simulink model "VSC_Simulink"  (R2019b)
settings: Solver=FixedStepDiscrete  StartTime=0.0  StopTime=Inf  FixedStep=T_pwm  MaxStep=1e-4  EnableMultiTasking=on
model workspace (MAT data in the model file):
  Control_P = 0
  Control_PI = 0
  I_integral = 0
  Id_pulse = 0
  Id_ref_const = 0
  Id_simulink = 0
  Id_sin = 0
  Iq_pulse = 0
  Iq_ref_const = 0
  Iq_simulink = 0
  Iq_sin = 0
  K_integral = 0
  K_proporcional = 0
  SELDACB = 0
  SELPWM4A = 0
  SELPWM4B = 0
  SELPWM5A = 0
  SELPWM5B = 0
  SELPWM6A = 0
  SELPWM6B = 0
  a_d = 0
  a_q = 0
  b_integral = 0
  b_proporcional = 0
  open = 0
  open_Id = 0
  open_Iq = 0
  open_control = 0
values from neighbouring files (symbols this model uses):
  Dec = 1    [Sotfware_Matlab.m]
  Frecuencia_Red = 50    [Sotfware_Matlab.m]
  Ib = 2.5    [Sotfware_Matlab.m]
  Ireg_PI = tan((90 + Fc_pi)*pi/180)/wo_pi    [Sotfware_Matlab.m]
  Kreg_P = 1/AP    [Sotfware_Matlab.m]
  Kreg_PI = Ac_pi*Ireg_PI*wo_pi / sqrt(1 + (Ireg_PI*wo_pi)^2)    [Sotfware_Matlab.m]
  Lpu = X_ind/ Lb    [Sotfware_Matlab.m]
  T_pwm = 1/Freq_Conmutacion    (= 0.0001)    [Sotfware_Matlab.m]
  TimerPeriod = Freq_Clock/(Freq_Conmutacion*4)    (= 5000)    [Sotfware_Matlab.m]
  Ub = 0.61*Vdc / sqrt(3)    [Sotfware_Matlab.m]
  w1pu = 1    [Sotfware_Matlab.m]
undefined symbols (not defined in the file or in its folder): Down, GPTRIP1SEL, GPTRIP2SEL, TZ1, TZ2, Up
libraries: c2802xlib x12, c2837xDlib x10, eeTransforms x2, simulink x2
(part 1 of 2)
settings Model: SimulationMode=external  ExtModeTrigDuration=8  TunableVars=SELPWM4A,SELPWM4B  TunableVarsStorageClass=Auto,Auto  TunableVarsTypeQualifier=const,const  ParameterArgumentNames=Control_P,Control_PI,I_integral,Id_pulse,Id_ref_const,Id_simulink,Id_sin,Iq_pulse,Iq_ref_const,Iq_simulink,Iq_sin,K_integral,K_proporcional,SELDACB,SELPWM4A,SELPWM4B,SELPWM5A,SELPWM5B,SELPWM6A,SELPWM6B,a_d,a_q,b_integral,b_proporcional,open,open_Id,open_Iq,open_control  OrderedModelArguments=off  Creator=jorge  LastModifiedBy=jorge
settings OptimizationCC: DefaultUnderspecifiedDataType=single  EnhancedBackFolding=on  PassReuseOutputArgsAs=Individual arguments  MaxStackSize=512  OptimizeBlockOrder=speed  DifferentSizesBufferReuse=on  OptimizationCustomize=off  EfficientTunableParamExpr=on
settings DebuggingCC: ParameterTunabilityLossMsg=error
settings HardwareCC: ProdBitPerChar=16  ProdBitPerInt=16  ProdBitPerPointer=32  ProdBitPerSizeT=32  ProdBitPerPtrDiffT=32  ProdLargestAtomicInteger=Integer  ProdLargestAtomicFloat=None  ProdWordSize=16  ProdLongLongMode=on  ProdHWDeviceType=Texas Instruments->C2000
settings SFSimCC: MATLABDynamicMemAlloc=off  CustomCodeUndefinedFunction=UseInterfaceOnly
settings RTWCC: SystemTargetFile=ert.tlc  HardwareBoard=TI Delfino F28379D LaunchPad  TLCOptions=-aInlineSetEventsForThisBaseRateFcn=TLC_FALSE -aSuppressMultiTaskScheduler=TLC_FALSE -aRateBasedStepFcn=1  TemplateMakefile=ert_default_tmf  GenerateReport=on  Toolchain=Texas Instruments Code Composer Studio (C2000)  IncludeHyperlinkInReport=on  LaunchReport=on  GenerateTraceInfo=on  GenerateTraceReport=on  GenerateTraceReportSl=on  GenerateTraceReportSf=on  GenerateTraceReportEml=on
settings CodeAppCC: ForceParamTrailComments=on  IgnoreCustomStorageClasses=off  OperatorAnnotations=on  SimulinkDataObjDesc=on  SFDataObjDesc=on  InsertBlockDesc=on
settings ERTTargetCC: CodeReplacementLibrary=TI C28x  SupportContinuousTime=on

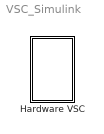
== system VSC_Simulink ==
  Hardware VSC : Subsystem  mask{Parameter1A=Id, Parameter1B=Id Referencia, Parameter2A=Iq, Parameter2B=Iq Referencia, ParameterDAC=Ángulo transformada de Park, Parameter3A=Va, Parameter3B=Ia, Id_simulink=1, Iq_simulink=1, refd=Pulsos, refq=Pulsos, control=Control PI, K_proporcional=Kreg_P, b_proporcional=1, K_integral=Kreg_PI*0.1, I_integral=Ireg_PI, b_integral=1, tipolazo=Lazo Cerrado, mandod=0, mandoq=0, acoplamiento=on}
      mask prompts: Parameter1A "PWM1A"; Parameter1B "PWM1B"; Parameter2A "PWM2A"; Parameter2B "PWM2B"; ParameterDAC "DAC - A"; Parameter3A "PWM3A"; Parameter3B "PWM3B"; Id_simulink "Id Referencia"; Iq_simulink "Iq Referencia"; refd "Forma de onda de referencia Id"; refq "Forma de onda de referencia Iq"; control "Selecciona el Control"; K_proporcional "K:"; b_proporcional "b:"; K_integral "K:"; I_integral "I:"; b_integral "b:"; tipolazo "Tipo de lazo"; mandod "Tensión de mando eje d  (md)"; mandoq "Tensión de mando eje q (mq)"
      mask init:
      | switch Parameter1A
      |     case 1
      |         SELPWM1A = 1;
      |     case 2
      |         SELPWM1A = 2;
      |     case 3
      |         SELPWM1A = 3;
      |     case 4
      |         SELPWM1A = 4;
      |     case 5
      |         SELPWM1A = 5;
      |     case 6
      |         SELPWM1A = 6;
      |     case 7
      |         SELPWM1A = 7;
      |     otherwise
      |         SELPWM1A = -1;
      | end
      | 
      | switch Parameter1B
      |     case 1
      |         SELPWM1B = 1;
      |     case 2
      |         SELPWM1B = 2;
      |     case 3
      |         SELPWM1B = 3;
      |     case 4
      |         SELPWM1B = 4;
      |     case 5
      |         SELPWM1B = 5;
      |     case 6
      |         SELPWM1B = 6;
      |     case 7
      |         SELPWM1B = 7;
      |     otherwise
      |         SELPWM1B = -1;
      | end
      | switch Parameter2A
      |     case 1
      |         SELPWM2A = 1;
      |     case 2
      |         SELPWM2A = 2;
      |     case 3
      |         SELPWM2A = 3;
      |     case 4
      |         SELPWM2A = 4;
      |     case 5
      |         SELPWM2A = 5;
      |     case 6
      |         SELPWM2A = 6;
      |     case 7
      |         SELPWM2A = 7;
      |     otherwise
      |         SELPWM2A = -1;
      | end
      | 
      | switch Parameter2B
      |     case 1
      |         SELPWM2B = 1;
      |     case 2
      |         SELPWM2B = 2;
      |     case 3
      |         SELPWM2B = 3;
      |     case 4
      |         SELPWM2B = 4;
      |     case 5
      |         SELPWM2B = 5;
      |     case 6
      |         SELPWM2B = 6;
      |     case 7
      |         SELPWM2B = 7;
      |     otherwise
      |         SELPWM2B = -1;
      | end
      | 
      | switch ParameterDAC
      |     case 1
      |         SELDACA = 1;
      |     case 2
      |         SELDACA = 2;
      |     case 3
      |         SELDACA = 3;
      |     case 4
      |         SELDACA = 4;
      |     case 5
      |         SELDACA = 5;
      |     case 6
      |         SELDACA = 6;
      |     case 7
      |         SELDACA = 7;
      |     otherwise
      |         SELDACA = -1;
      | end
      | switch Parameter3A
      |     case 1
      |         SELPWM3A = 8;
      |     case 2
      |         SELPWM3A = 9;
      |     case 3
      |         SELPWM3A = 10;
      |     case 4
      |         SELPWM3A = 11;
      |     case 5
      |         SELPWM3A = 12;
      |     case 6
      |         SELPWM3A = 13;
      |     otherwise
      |         SELPWM3A = -1;
      | end
      | switch Parameter3B
      |     case 1
      |         SELPWM3B = 8;
      |     case 2
      |         SELPWM3B = 9;
      |     case 3
      |         SELPWM3B = 10;
      |     case 4
      |         SELPWM3B = 11;
      |     case 5
      |         SELPWM3B = 12;
      |     case 6
      |         SELPWM3B = 13;
      |     otherwise
      |         SELPWM3B = -1;
      | end
      |        
      | switch refd
      |     case 1
      |         Id_ref_const = 1;
      |         Id_pulse = 0;
      |         Id_sin = 0;
      |     case 2
      |         Id_ref_const = 0;
      |         Id_pulse = 1;
      |         Id_sin = 0;        
      |     case 3
      |         Id_ref_const = 0;
      |         Id_pulse = 0;
      |         Id_sin = 1;
      | end
      | 
      | switch refq
      |     case 1
      |         Iq_ref_const = 1;
      |         Iq_pulse = 0;
      |         Iq_sin = 0;
      |     case 2
      |         Iq_ref_const = 0;
      |         Iq_pulse = 1;
      |         Iq_sin = 0;        
      |     case 3
      |         Iq_ref_const = 0;
      |         Iq_pulse = 0;
      |         Iq_sin = 1;
      | end
      | 
      | switch control
      |     case 1
      |         Control_P = 1;
      |         Control_PI = 0;
      |         I_integral = 1;
      |     case 2
      |         Control_P = 0;
      |         Control_PI = 1;
      | end
      | 
      | switch tipolazo
      |     case 1
      |         open = 0;
      |         a_d = mandod;
      |         a_q = mandoq;
      |     case 2
      |         open = 1;
      |         a_d = 0;
      |         a_q = 0;
      | end
      | 
      | if acoplamiento == 1
      |         open_Id = 1;
      |         open_Iq = 1;
      | else 
      |     open_Id = 0;
      |     open_Iq = 0;
      | end
      mask TypeOptions Parameter1A: Id | Iq | Id Referencia | Iq Referencia | md | mq | Ángulo transformada de Park
      mask TypeOptions Parameter1B: Id | Iq | Id Referencia | Iq Referencia | md | mq | Ángulo transformada de Park
      mask TypeOptions Parameter2A: Id | Iq | Id Referencia | Iq Referencia | md | mq | Ángulo transformada de Park
      mask TypeOptions Parameter2B: Id | Iq | Id Referencia | Iq Referencia | md | mq | Ángulo transformada de Park
      mask TypeOptions ParameterDAC: Id | Iq | Id Referencia | Iq Referencia | md | mq | Ángulo transformada de Park
      mask TypeOptions Parameter3A: Va | Vb | Vc | Ia | Ib | Ic
      mask TypeOptions Parameter3B: Va | Vb | Vc | Ia | Ib | Ic
      mask TypeOptions refd: Constante | Pulsos | Senoidal
      mask TypeOptions refq: Constante | Pulsos | Senoidal
      mask TypeOptions control: Control P | Control PI
      mask TypeOptions tipolazo: Lazo Abierto | Lazo Cerrado
      mask DialogControl Container7 Prompt: Salidas
      mask DialogControl Container9 Prompt: Referencias
      mask DialogControl Container12 Prompt: Controles
      mask DialogControl Container22 Prompt: Control Proporcional
      mask DialogControl Container24 Prompt: Control Proporcional - Integral
      mask DialogControl Container19 Prompt: Lazo
      mask DialogControl Container17 Prompt: Lazo Abierto
      mask DialogControl Container18 Prompt: Acoplamiento / Desacoplamiento
      mask Display: image('click.png'); % Use "Edit Image" on toolstrip to change.

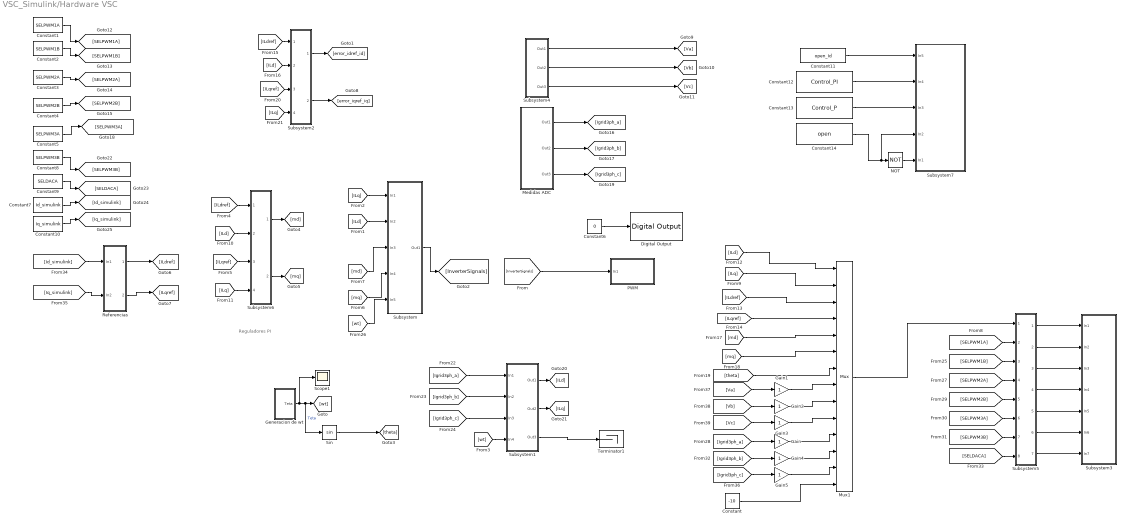
== system VSC_Simulink/Hardware VSC ==
  note: Reguladores PI
  Constant : Constant  Value=-10
  Constant1 : Constant  Value=SELPWM1A  SampleTime=-1
  Constant10 : Constant  Value=Iq_simulink  SampleTime=-1
  Constant11 : Constant  Value=open_Id  OutDataTypeStr=uint16  SampleTime=-1
  Constant12 : Constant  Value=Control_PI  SampleTime=-1
  Constant13 : Constant  Value=Control_P  SampleTime=-1
  Constant14 : Constant  Value=open  SampleTime=-1
  Constant2 : Constant  Value=SELPWM1B  SampleTime=-1
  Constant3 : Constant  Value=SELPWM2A  SampleTime=-1
  Constant4 : Constant  Value=SELPWM2B  SampleTime=-1
  Constant5 : Constant  Value=SELPWM3A
  Constant6 : Constant  Value=0  OutDataTypeStr=uint16  SampleTime=-1
  Constant7 : Constant  Value=Id_simulink  SampleTime=-1
  Constant8 : Constant  Value=SELPWM3B  SampleTime=-1
  Constant9 : Constant  Value=SELDACA  SampleTime=-1
  Digital Output : c2837xDlib/Digital Output  GPIO_Number=GPIO24~GPIO31  GPIO_Bit0=off  GPIO_BIT0_Toggle=off  GPIO_Bit1=off  GPIO_BIT1_Toggle=off  GPIO_Bit2=on  GPIO_BIT2_Toggle=on  GPIO_Bit3=off  GPIO_BIT3_Toggle=off  GPIO_Bit4=off  GPIO_BIT4_Toggle=off  GPIO_Bit5=off  GPIO_BIT5_Toggle=off  GPIO_Bit6=off  GPIO_BIT6_Toggle=off  GPIO_Bit7=off  GPIO_BIT7_Toggle=off
      settings: SourceProductName=Embedded Coder Support Package for Texas Instruments C2000 Processors  SourceProductBaseCode=TIC2000
  Gain{,1..5} (6 alike) : Gain  OutDataTypeStr=double
  Generacion de wt : Subsystem
  Medidas ADC : Subsystem
  Mux1 : Mux  Inputs=14
  NOT : Logic  Operator=NOT  IconShape=distinctive  AllPortsSameDT=off  OutDataTypeStr=boolean
  PWM : Subsystem
  Referencias : Subsystem
  Scope1 : Scope
  Sin : Trigonometry
  Subsystem : Subsystem
  Subsystem1 : Subsystem
  Subsystem2 : Subsystem
  Subsystem3 : Subsystem
  Subsystem4 : Subsystem
  Subsystem5 : Subsystem
  Subsystem6 : Subsystem
  Subsystem7 : Subsystem
  Terminator1 : Terminator
  wires:
  [Iq_simulink] -> Referencias/2(In2)
  [Id_simulink] -> Referencias/1(In1)
  Constant10/1 -> [Iq_simulink]
  Constant7/1 -> [Id_simulink]
  Constant9/1 -> [SELDACA]
  Constant4/1 -> [SELPWM2B]
  Constant5/1 -> [SELPWM3A]
  Constant3/1 -> [SELPWM2A]
  Constant2/1 -> [SELPWM1B]
  Constant1/1 -> [SELPWM1A]
  [SELDACA] -> Subsystem5/8(In8)
  [SELPWM3A] -> Subsystem5/6(In6)
  [SELPWM2B] -> Subsystem5/5(In5)
  [SELPWM2A] -> Subsystem5/4(In4)
  [SELPWM1B] -> Subsystem5/3(In3)
  [SELPWM1A] -> Subsystem5/2(In2)
  Mux1/1 -> Subsystem5/1(In1)
  Subsystem5/7(Out6) -> Subsystem3/7(In7)
  Subsystem5/6(Out5) -> Subsystem3/6(In6)
  Subsystem5/5(Out4) -> Subsystem3/5(In5)
  Subsystem5/4(Out3) -> Subsystem3/4(In4)
  Subsystem5/3(Out2) -> Subsystem3/3(In3)
  Subsystem5/2(Out1) -> Subsystem3/2(In2)
  Subsystem5/1(Out7) -> Subsystem3/1(In1)
  [md] -> Mux1/5
  [ILq] -> Mux1/2
  [ILd] -> Mux1/1
  [ILqref] -> Mux1/4
  [ILdref] -> Mux1/3
  Subsystem4/3(Out3) -> [Vc]
  Subsystem4/2(Out2) -> [Vb]
  Subsystem4/1(Out1) -> [Va]
  Constant6/1 -> Digital Output/1
  Subsystem2/2(Out2) -> [error_iqref_iq]
  Subsystem2/1(Out1) -> [error_idref_id]
  [ILq] -> Subsystem2/4(In4)
  [ILqref] -> Subsystem2/3(In3)
  [ILd] -> Subsystem2/2(In2)
  [ILdref] -> Subsystem2/1(In1)
  Sin/1 -> [theta]
  [md] -> Subsystem/3(In3)
  [mq] -> Subsystem/4(In4)
  Subsystem1/3(Out3) -> Terminator1/1
  Subsystem1/2(Out2) -> [ILq]
  [wt] -> Subsystem1/4(In4)
  [Igrid3ph_c] -> Subsystem1/3(In3)
  [Igrid3ph_b] -> Subsystem1/2(In2)
  [Igrid3ph_a] -> Subsystem1/1(In1)
  Subsystem1/1(Out1) -> [ILd]
  Referencias/2(Out2) -> [ILqref]
  Referencias/1(Out1) -> [ILdref]
  Subsystem/1(Out1) -> [InverterSignals]
  [wt] -> Subsystem/5(In5)
  [ILd] -> Subsystem/2(In2)
  [ILq] -> Subsystem/1(In1)
  Medidas ADC/3(Out3) -> [Igrid3ph_c]
  Medidas ADC/2(Out2) -> [Igrid3ph_b]
  Medidas ADC/1(Out1) -> [Igrid3ph_a]
  [InverterSignals] -> PWM/1(In1)
  Generacion de wt/1(Teta) -> Scope1/1, [wt], Sin/1  "Teta"
  Constant8/1 -> [SELPWM3B]
  [mq] -> Mux1/6
  [theta] -> Mux1/7
  [Igrid3ph_a] -> Gain/1
  Gain/1 -> Mux1/11
  Gain4/1 -> Mux1/12
  [Igrid3ph_b] -> Gain4/1
  [Igrid3ph_c] -> Gain5/1
  Gain5/1 -> Mux1/13
  [Vc] -> Gain3/1
  [Vb] -> Gain2/1
  [Va] -> Gain1/1
  Gain1/1 -> Mux1/8
  Gain2/1 -> Mux1/9
  Gain3/1 -> Mux1/10
  Constant/1 -> Mux1/14
  [SELPWM3B] -> Subsystem5/7(In7)
  Constant14/1 -> Subsystem7/4(In2), NOT/1
  Subsystem6/2(Out2) -> [mq]
  [ILdref] -> Subsystem6/1(In1)
  [ILqref] -> Subsystem6/3(In3)
  [ILq] -> Subsystem6/4(In4)
  [ILd] -> Subsystem6/2(In2)
  Subsystem6/1(Out1) -> [md]
  Constant13/1 -> Subsystem7/3(In3)
  Constant12/1 -> Subsystem7/2(In4)
  Constant11/1 -> Subsystem7/1(In5)
  NOT/1 -> Subsystem7/5(In1)

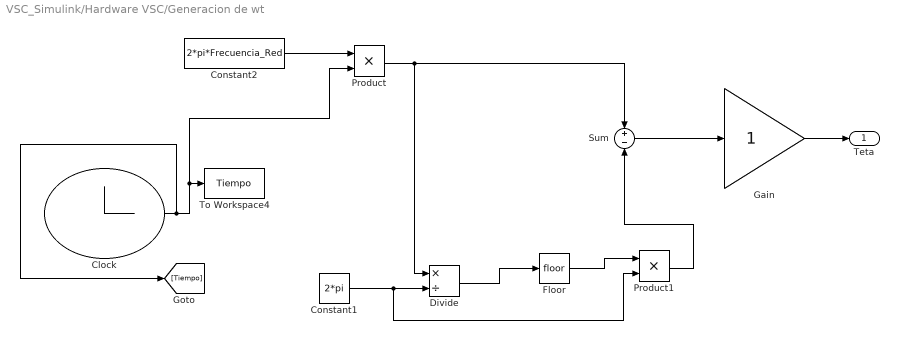
== system VSC_Simulink/Hardware VSC/Generacion de wt ==
  Clock : Clock
      settings: Decimation=100
  Constant1 : Constant  Value=2*pi  SampleTime=-1
  Constant2 : Constant  Value=2*pi*Frecuencia_Red  SampleTime=-1
  Divide : Product  Inputs=*/
  Floor : Rounding
  Gain : Gain
  Product : Product
  Product1 : Product
  Sum : Sum  Inputs=+-
  To Workspace4 : ToWorkspace  VariableName=Tiempo
  Teta : Outport  VectorParamsAs1DForOutWhenUnconnected=off
  wires:
  Product/1 -> Sum/1, Divide/1
  Constant1/1 -> Divide/2, Product1/2
  Product1/1 -> Sum/2
  Sum/1 -> Gain/1
  Divide/1 -> Floor/1
  Floor/1 -> Product1/1
  Constant2/1 -> Product/1
  Clock/1 -> To Workspace4/1, Product/2, [Tiempo]
  Gain/1 -> Teta/1

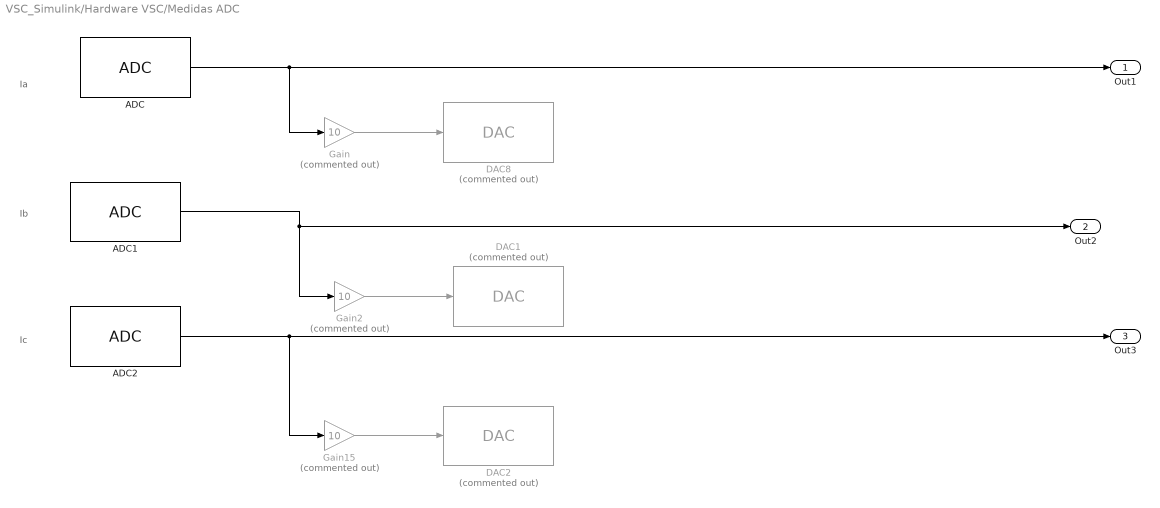
== system VSC_Simulink/Hardware VSC/Medidas ADC ==
  note: Ic
  note: Ia
  note: Ib
  ADC : c2802xlib/ADC  blkParamProc=C2000_Type4  ADCModule=C  samplingMode=Single sample mode  ADCResolution=12-bit (Single-ended input)  useSOC1=SOC8  useSOC2=SOC0_SOC1  SOCAcquisitionWindow=15  SOCTriggerSource=ePWM4_ADCSOCA  SOCInterruptTrigger=No ADCINT  Ts=-1  dType=uint16  postInterrupt=on  interruptSel=ADCINT1  ADCINTContinuous=on  endma=off  chdma=1  conv1=ADCINA0  conv2=ADCINA0 and ADCINB0  conv1_Type4=ADCIN4  conv2_Type4=ADCIN0 and ADCIN1
      settings: SourceProductName=Embedded Coder Support Package for Texas Instruments C2000 Processors
  ADC1 : c2802xlib/ADC  blkParamProc=C2000_Type4  ADCModule=B  samplingMode=Single sample mode  ADCResolution=12-bit (Single-ended input)  useSOC1=SOC9  useSOC2=SOC0_SOC1  SOCAcquisitionWindow=15  SOCTriggerSource=ePWM5_ADCSOCA  SOCInterruptTrigger=No ADCINT  Ts=-1  dType=uint16  postInterrupt=on  interruptSel=ADCINT1  ADCINTContinuous=on  endma=off  chdma=1  conv1=ADCINA0  conv2=ADCINA0 and ADCINB0  conv1_Type4=ADCIN4  conv2_Type4=ADCIN0 and ADCIN1
      settings: SourceProductName=Embedded Coder Support Package for Texas Instruments C2000 Processors
  ADC2 : c2802xlib/ADC  blkParamProc=C2000_Type4  ADCModule=A  samplingMode=Single sample mode  ADCResolution=12-bit (Single-ended input)  useSOC1=SOC10  useSOC2=SOC0_SOC1  SOCAcquisitionWindow=15  SOCTriggerSource=ePWM6_ADCSOCA  SOCInterruptTrigger=No ADCINT  Ts=-1  dType=uint16  postInterrupt=on  interruptSel=ADCINT1  ADCINTContinuous=on  endma=off  chdma=1  conv1=ADCINA0  conv2=ADCINA0 and ADCINB0  conv1_Type4=ADCIN4  conv2_Type4=ADCIN0 and ADCIN1
      settings: SourceProductName=Embedded Coder Support Package for Texas Instruments C2000 Processors
  DAC1 : c2837xDlib/DAC  Commented=on  channel=B  saturate=off
      settings: SourceProductName=Embedded Coder Support Package for Texas Instruments C2000 Processors  SourceProductBaseCode=TIC2000
  DAC2 : c2837xDlib/DAC  Commented=on  channel=B  saturate=off
      settings: SourceProductName=Embedded Coder Support Package for Texas Instruments C2000 Processors  SourceProductBaseCode=TIC2000
  DAC8 : c2837xDlib/DAC  Commented=on  channel=B  saturate=off
      settings: SourceProductName=Embedded Coder Support Package for Texas Instruments C2000 Processors  SourceProductBaseCode=TIC2000
  Gain : Gain  Commented=on  Gain=10
  Gain15 : Gain  Commented=on  Gain=10
  Gain2 : Gain  Commented=on  Gain=10
  Out1 : Outport  VectorParamsAs1DForOutWhenUnconnected=off
  Out2 : Outport  Port=2  VectorParamsAs1DForOutWhenUnconnected=off
  Out3 : Outport  Port=3  VectorParamsAs1DForOutWhenUnconnected=off
  wires:
  Gain/1 -> DAC8/1
  ADC2/1 -> Gain15/1, Out3/1
  ADC1/1 -> Gain2/1, Out2/1
  Gain2/1 -> DAC1/1
  Gain15/1 -> DAC2/1
  ADC/1 -> Gain/1, Out1/1

== system VSC_Simulink/Hardware VSC/PWM ==
  In1 : Inport
  Demux2 : Demux  Outputs=3
  ePWM1 : c2802xlib/ePWM  useModule=ePWM5  ePWMxLINKTBPRD=Not Linked  periodUnits=Clock cycles  timerSource=Specify via dialog  timerPeriod_clk=TimerPeriod  timerPeriod_sec=0.0001  tbshadow=Counter equals to zero  countingMode=Up-Down  phaseActiveEnable=Disable  phaseDirection=Count down after sync  phaseActive=0  synchronizationEnable=off  dcaevt1Sync=off  dcbevt1Sync=off  synchronizationOption=Disable  clockPrescale=1  HSclockPrescale=1  enswap=off  ePWMxAStatus=on  ePWMxAactionLogic1=Set  ePWMxAactionLogic2=Clear  ePWMxAactionLogic3=Clear  ePWMxAactionLogic4=Set  ePWMxAactionLogic5=Do nothing  ePWMxAactionLogic6=Do nothing  ePWMxALoadMode=Load on counter equals to zero (CTR=Zero)  ePWMxACSFenable=off  ePWMxACSFvalue=Forcing disable  ePWMxASFreload=Zero  ePWMxBStatus=off  ePWMxBactionLogic1=Set  ePWMxBactionLogic2=Clear  ePWMxBactionLogic3=Do nothing  ePWMxBactionLogic4=Do nothing  ePWMxBactionLogic5=Clear  ePWMxBactionLogic6=Set  ePWMxBLoadMode=Load on counter equals to zero (CTR=Zero)  ePWMxBCSFenable=off  ePWMxBCSFvalue=Forcing disable  ePWMxBSFreload=Zero  ePWNxBOutWay=off  ePWMxLINKCMPA=Not Linked  CMPAUnits=Clock cycles  CMPASource=Input port  CMPAValue_per=50  CMPAValue_clk=0  enCMPAshadow=Counter equals to zero  ePWMxLINKCMPB=Not Linked  CMPBUnits=Clock cycles  CMPBSource=Specify via dialog  CMPBValue_per=50  CMPBValue_clk=0  enCMPBshadow=Counter equals to zero  ePWMxLINKCMPC=Not Linked  CMPCUnits=Clock cycles  CMPCSource=Specify via dialog  CMPCValue_per=50  CMPCValue_clk=0  enCMPCshadow=Counter equals to zero  ePWMxLINKCMPD=Not Linked  CMPDUnits=Clock cycles  CMPDSource=Specify via dialog  CMPDValue_per=50  CMPDValue_clk=0  enCMPDshadow=Counter equals to zero  enableDBePWMxA=off  enableDBePWMxB=on  enhalfcycle=off  DBpolarity=Active high (AH)  DBedgeDelay=Negative  DBSource_ePWMxA=ePWMxA  DBSource_ePWMxB=ePWMxA  DBperiodSource=Specify via dialog  REDperiod=0  FEDperiod=0  adcstartModuleA=on  adcrequestEventA=Third event  adcstartEventA=Digital Compare Module A Event 1 start of conversion (DCAEVT1.soc)  adcstartEventA_type2=Counter equals to period (CTR=PRD)  adcstartModuleB=on  adcrequestEventB=Third event  adcstartEventB=Counter equals to zero (CTR=Zero)  adcstartEventB_type2=Counter equals to period (CTR=PRD)  intEn=off  intPrd=First event  intSel=Counter equals to zero (CTR=Zero)  intSel_type2=Counter equals to zero (CTR=Zero)  hrpe=off  enHRPWM=off  HRPWM_LoadMode=Counter equals to period (CTR=PRD)  HRPWM_CTLMode=Duty or Period control mode  HRPWM_EDGMode=Both edge  hrpeb=off  enHRPWMB=off  HRPWM_LoadModeB=Counter equals to zero (CTR=ZERO)  HRPWM_CTLModeB=Duty or Period control mode  HRPWM_EDGModeB=Both edge  enSFO=on  enautoconv=on  chopperEnable=off  chopperFrequency=1  chopperFirstwidth=1  chopperDuty=12.5%  tripZonesource=Specify via dialog  tzselOSHT1=off  tzselOSHT2=off  tzselOSHT3=off  tzselOSHDCAEV1=off  tzselOSHDCBEV1=off  tzselCBC1=off  tzselCBC2=off  tzselCBC3=off  tzselCBCDCAEV2=off  tzselCBCDCBEV2=off  tzselOSHT4=off  tzselOSHT5=off  tzselOSHT6=off  tzselCBC4=off  tzselCBC5=off  tzselCBC6=off  enTzOstIntr=off  enTzCbcIntr=off  enTzDCAEVT1Intr=off  enTzDCAEVT2Intr=off  enTzDCBEVT1Intr=off  enTzDCBEVT2Intr=off  ePWMxAforced=No action  ePWMxBforced=No action  DCAEVT1forced=No action  DCBEVT1forced=No action  DCAEVT2forced=No action  DCBEVT2forced=No action  dcah=Trip Zone 1 input (TZ1)  dcal=Trip Zone 2 input (TZ2)  dcbh=Trip Zone 1 input (TZ1)  dcbl=Trip Zone 2 input (TZ2)  dcah_type2=GPTRIP1SEL/(TZ1)  dcal_type2=GPTRIP2SEL/(TZ2)  dcbh_type2=GPTRIP1SEL/(TZ1)  dcbl_type2=GPTRIP2SEL/(TZ2)  gendcaevt1=Event disabled  gendcaevt2=Event disabled  gendcbevt1=Event disabled  gendcbevt2=Event disabled  dcaevt1src=DCAEVT1 with sync  dcaevt2src=DCAEVT2 with sync  dcbevt1src=DCBEVT1 with sync  dcbevt2src=DCBEVT2 with sync  pulsesel=Counter equals to zero (CTR=Zero)  blankinv=off  blankoffset=0  blankwidth=0  evsrcsel=Filtered version of DCAEVT1 (DCAEVT1FILT)  encape=off  PwmType=C2000_Type4
      settings: SourceProductName=Embedded Coder Support Package for Texas Instruments C2000 Processors
  ePWM2 : c2802xlib/ePWM  useModule=ePWM6  ePWMxLINKTBPRD=Not Linked  periodUnits=Clock cycles  timerSource=Specify via dialog  timerPeriod_clk=TimerPeriod  timerPeriod_sec=0.0001  tbshadow=Counter equals to zero  countingMode=Up-Down  phaseActiveEnable=Disable  phaseDirection=Count down after sync  phaseActive=0  synchronizationEnable=off  dcaevt1Sync=off  dcbevt1Sync=off  synchronizationOption=Disable  clockPrescale=1  HSclockPrescale=1  enswap=off  ePWMxAStatus=on  ePWMxAactionLogic1=Set  ePWMxAactionLogic2=Clear  ePWMxAactionLogic3=Clear  ePWMxAactionLogic4=Set  ePWMxAactionLogic5=Do nothing  ePWMxAactionLogic6=Do nothing  ePWMxALoadMode=Load on counter equals to zero (CTR=Zero)  ePWMxACSFenable=off  ePWMxACSFvalue=Forcing disable  ePWMxASFreload=Zero  ePWMxBStatus=off  ePWMxBactionLogic1=Set  ePWMxBactionLogic2=Clear  ePWMxBactionLogic3=Do nothing  ePWMxBactionLogic4=Do nothing  ePWMxBactionLogic5=Clear  ePWMxBactionLogic6=Set  ePWMxBLoadMode=Load on counter equals to zero (CTR=Zero)  ePWMxBCSFenable=off  ePWMxBCSFvalue=Forcing disable  ePWMxBSFreload=Zero  ePWNxBOutWay=off  ePWMxLINKCMPA=Not Linked  CMPAUnits=Clock cycles  CMPASource=Input port  CMPAValue_per=50  CMPAValue_clk=0  enCMPAshadow=Counter equals to zero  ePWMxLINKCMPB=Not Linked  CMPBUnits=Clock cycles  CMPBSource=Specify via dialog  CMPBValue_per=50  CMPBValue_clk=0  enCMPBshadow=Counter equals to zero  ePWMxLINKCMPC=Not Linked  CMPCUnits=Clock cycles  CMPCSource=Specify via dialog  CMPCValue_per=50  CMPCValue_clk=0  enCMPCshadow=Counter equals to zero  ePWMxLINKCMPD=Not Linked  CMPDUnits=Clock cycles  CMPDSource=Specify via dialog  CMPDValue_per=50  CMPDValue_clk=0  enCMPDshadow=Counter equals to zero  enableDBePWMxA=off  enableDBePWMxB=on  enhalfcycle=off  DBpolarity=Active high (AH)  DBedgeDelay=Negative  DBSource_ePWMxA=ePWMxA  DBSource_ePWMxB=ePWMxA  DBperiodSource=Specify via dialog  REDperiod=0  FEDperiod=0  adcstartModuleA=on  adcrequestEventA=Third event  adcstartEventA=Digital Compare Module A Event 1 start of conversion (DCAEVT1.soc)  adcstartEventA_type2=Counter equals to period (CTR=PRD)  adcstartModuleB=on  adcrequestEventB=Third event  adcstartEventB=Counter equals to zero (CTR=Zero)  adcstartEventB_type2=Counter equals to period (CTR=PRD)  intEn=off  intPrd=First event  intSel=Counter equals to zero (CTR=Zero)  intSel_type2=Counter equals to zero (CTR=Zero)  hrpe=off  enHRPWM=off  HRPWM_LoadMode=Counter equals to period (CTR=PRD)  HRPWM_CTLMode=Duty or Period control mode  HRPWM_EDGMode=Both edge  hrpeb=off  enHRPWMB=off  HRPWM_LoadModeB=Counter equals to zero (CTR=ZERO)  HRPWM_CTLModeB=Duty or Period control mode  HRPWM_EDGModeB=Both edge  enSFO=on  enautoconv=on  chopperEnable=off  chopperFrequency=1  chopperFirstwidth=1  chopperDuty=12.5%  tripZonesource=Specify via dialog  tzselOSHT1=off  tzselOSHT2=off  tzselOSHT3=off  tzselOSHDCAEV1=off  tzselOSHDCBEV1=off  tzselCBC1=off  tzselCBC2=off  tzselCBC3=off  tzselCBCDCAEV2=off  tzselCBCDCBEV2=off  tzselOSHT4=off  tzselOSHT5=off  tzselOSHT6=off  tzselCBC4=off  tzselCBC5=off  tzselCBC6=off  enTzOstIntr=off  enTzCbcIntr=off  enTzDCAEVT1Intr=off  enTzDCAEVT2Intr=off  enTzDCBEVT1Intr=off  enTzDCBEVT2Intr=off  ePWMxAforced=No action  ePWMxBforced=No action  DCAEVT1forced=No action  DCBEVT1forced=No action  DCAEVT2forced=No action  DCBEVT2forced=No action  dcah=Trip Zone 1 input (TZ1)  dcal=Trip Zone 2 input (TZ2)  dcbh=Trip Zone 1 input (TZ1)  dcbl=Trip Zone 2 input (TZ2)  dcah_type2=GPTRIP1SEL/(TZ1)  dcal_type2=GPTRIP2SEL/(TZ2)  dcbh_type2=GPTRIP1SEL/(TZ1)  dcbl_type2=GPTRIP2SEL/(TZ2)  gendcaevt1=Event disabled  gendcaevt2=Event disabled  gendcbevt1=Event disabled  gendcbevt2=Event disabled  dcaevt1src=DCAEVT1 with sync  dcaevt2src=DCAEVT2 with sync  dcbevt1src=DCBEVT1 with sync  dcbevt2src=DCBEVT2 with sync  pulsesel=Counter equals to zero (CTR=Zero)  blankinv=off  blankoffset=0  blankwidth=0  evsrcsel=Filtered version of DCAEVT1 (DCAEVT1FILT)  encape=off  PwmType=C2000_Type4
      settings: SourceProductName=Embedded Coder Support Package for Texas Instruments C2000 Processors
  ePWM3 : c2802xlib/ePWM  useModule=ePWM4  ePWMxLINKTBPRD=Not Linked  periodUnits=Clock cycles  timerSource=Specify via dialog  timerPeriod_clk=TimerPeriod  timerPeriod_sec=0.0001  tbshadow=Counter equals to zero  countingMode=Up-Down  phaseActiveEnable=Disable  phaseDirection=Count down after sync  phaseActive=0  synchronizationEnable=off  dcaevt1Sync=off  dcbevt1Sync=off  synchronizationOption=Disable  clockPrescale=1  HSclockPrescale=1  enswap=off  ePWMxAStatus=on  ePWMxAactionLogic1=Set  ePWMxAactionLogic2=Clear  ePWMxAactionLogic3=Clear  ePWMxAactionLogic4=Set  ePWMxAactionLogic5=Do nothing  ePWMxAactionLogic6=Do nothing  ePWMxALoadMode=Load on counter equals to zero (CTR=Zero)  ePWMxACSFenable=off  ePWMxACSFvalue=Forcing disable  ePWMxASFreload=Zero  ePWMxBStatus=off  ePWMxBactionLogic1=Set  ePWMxBactionLogic2=Clear  ePWMxBactionLogic3=Do nothing  ePWMxBactionLogic4=Do nothing  ePWMxBactionLogic5=Clear  ePWMxBactionLogic6=Set  ePWMxBLoadMode=Load on counter equals to zero (CTR=Zero)  ePWMxBCSFenable=off  ePWMxBCSFvalue=Forcing disable  ePWMxBSFreload=Zero  ePWNxBOutWay=off  ePWMxLINKCMPA=Not Linked  CMPAUnits=Clock cycles  CMPASource=Input port  CMPAValue_per=50  CMPAValue_clk=0  enCMPAshadow=Counter equals to zero  ePWMxLINKCMPB=Not Linked  CMPBUnits=Clock cycles  CMPBSource=Specify via dialog  CMPBValue_per=50  CMPBValue_clk=0  enCMPBshadow=Counter equals to zero  ePWMxLINKCMPC=Not Linked  CMPCUnits=Clock cycles  CMPCSource=Specify via dialog  CMPCValue_per=50  CMPCValue_clk=0  enCMPCshadow=Counter equals to zero  ePWMxLINKCMPD=Not Linked  CMPDUnits=Clock cycles  CMPDSource=Specify via dialog  CMPDValue_per=50  CMPDValue_clk=0  enCMPDshadow=Counter equals to zero  enableDBePWMxA=off  enableDBePWMxB=on  enhalfcycle=off  DBpolarity=Active high (AH)  DBedgeDelay=Negative  DBSource_ePWMxA=ePWMxA  DBSource_ePWMxB=ePWMxA  DBperiodSource=Specify via dialog  REDperiod=0  FEDperiod=0  adcstartModuleA=on  adcrequestEventA=Third event  adcstartEventA=Digital Compare Module A Event 1 start of conversion (DCAEVT1.soc)  adcstartEventA_type2=Counter equals to period (CTR=PRD)  adcstartModuleB=on  adcrequestEventB=Third event  adcstartEventB=Counter equals to zero (CTR=Zero)  adcstartEventB_type2=Counter equals to period (CTR=PRD)  intEn=off  intPrd=First event  intSel=Counter equals to zero (CTR=Zero)  intSel_type2=Counter equals to zero (CTR=Zero)  hrpe=off  enHRPWM=off  HRPWM_LoadMode=Counter equals to period (CTR=PRD)  HRPWM_CTLMode=Duty or Period control mode  HRPWM_EDGMode=Both edge  hrpeb=off  enHRPWMB=off  HRPWM_LoadModeB=Counter equals to zero (CTR=ZERO)  HRPWM_CTLModeB=Duty or Period control mode  HRPWM_EDGModeB=Both edge  enSFO=on  enautoconv=on  chopperEnable=off  chopperFrequency=1  chopperFirstwidth=1  chopperDuty=12.5%  tripZonesource=Specify via dialog  tzselOSHT1=off  tzselOSHT2=off  tzselOSHT3=off  tzselOSHDCAEV1=off  tzselOSHDCBEV1=off  tzselCBC1=off  tzselCBC2=off  tzselCBC3=off  tzselCBCDCAEV2=off  tzselCBCDCBEV2=off  tzselOSHT4=off  tzselOSHT5=off  tzselOSHT6=off  tzselCBC4=off  tzselCBC5=off  tzselCBC6=off  enTzOstIntr=off  enTzCbcIntr=off  enTzDCAEVT1Intr=off  enTzDCAEVT2Intr=off  enTzDCBEVT1Intr=off  enTzDCBEVT2Intr=off  ePWMxAforced=No action  ePWMxBforced=No action  DCAEVT1forced=No action  DCBEVT1forced=No action  DCAEVT2forced=No action  DCBEVT2forced=No action  dcah=Trip Zone 1 input (TZ1)  dcal=Trip Zone 2 input (TZ2)  dcbh=Trip Zone 1 input (TZ1)  dcbl=Trip Zone 2 input (TZ2)  dcah_type2=GPTRIP1SEL/(TZ1)  dcal_type2=GPTRIP2SEL/(TZ2)  dcbh_type2=GPTRIP1SEL/(TZ1)  dcbl_type2=GPTRIP2SEL/(TZ2)  gendcaevt1=Event disabled  gendcaevt2=Event disabled  gendcbevt1=Event disabled  gendcbevt2=Event disabled  dcaevt1src=DCAEVT1 with sync  dcaevt2src=DCAEVT2 with sync  dcbevt1src=DCBEVT1 with sync  dcbevt2src=DCBEVT2 with sync  pulsesel=Counter equals to zero (CTR=Zero)  blankinv=off  blankoffset=0  blankwidth=0  evsrcsel=Filtered version of DCAEVT1 (DCAEVT1FILT)  encape=off  PwmType=C2000_Type4
      settings: SourceProductName=Embedded Coder Support Package for Texas Instruments C2000 Processors
  wires:
  Demux2/2 -> ePWM1/1
  Demux2/3 -> ePWM2/1
  Demux2/1 -> ePWM3/1
  In1/1 -> Demux2/1

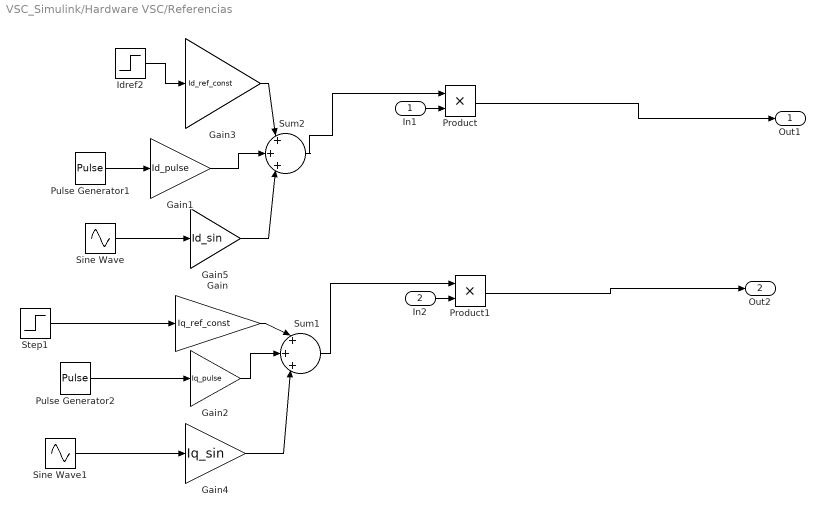
== system VSC_Simulink/Hardware VSC/Referencias ==
  In1 : Inport
  In2 : Inport  Port=2
  Gain : Gain  Gain=Iq_ref_const
  Gain1 : Gain  Gain=Id_pulse
  Gain2 : Gain  Gain=Iq_pulse
  Gain3 : Gain  Gain=Id_ref_const
  Gain4 : Gain  Gain=Iq_sin
  Gain5 : Gain  Gain=Id_sin
  Idref2 : Step  Time=0.3
  Product : Product
  Product1 : Product
  Pulse Generator1 : DiscretePulseGenerator  Period=100000  PulseWidth=100000*0.5  SampleTime=T_pwm  VectorParams1D=off
  Pulse Generator2 : DiscretePulseGenerator  Period=100000  PulseWidth=100000*0.5  PhaseDelay=100000*0.3  SampleTime=T_pwm  VectorParams1D=off
  Sine Wave : Sin  SineType=Sample based  Samples=10000  SampleTime=T_pwm
  Sine Wave1 : Sin  SineType=Sample based  Samples=10000  SampleTime=T_pwm
  Step1 : Step  Time=3
  Sum1 : Sum  Inputs=|+|+|+|
  Sum2 : Sum  Inputs=|+|+|+|
  Out1 : Outport  VectorParamsAs1DForOutWhenUnconnected=off
  Out2 : Outport  Port=2  VectorParamsAs1DForOutWhenUnconnected=off
  wires:
  In2/1 -> Product1/2
  In1/1 -> Product/2
  Product1/1 -> Out2/1
  Product/1 -> Out1/1
  Idref2/1 -> Gain3/1
  Pulse Generator1/1 -> Gain1/1
  Sum2/1 -> Product/1
  Sum1/1 -> Product1/1
  Pulse Generator2/1 -> Gain2/1
  Step1/1 -> Gain/1
  Gain/1 -> Sum1/1
  Gain3/1 -> Sum2/1
  Gain2/1 -> Sum1/2
  Gain1/1 -> Sum2/2
  Sine Wave/1 -> Gain5/1
  Sine Wave1/1 -> Gain4/1
  Gain4/1 -> Sum1/3
  Gain5/1 -> Sum2/3

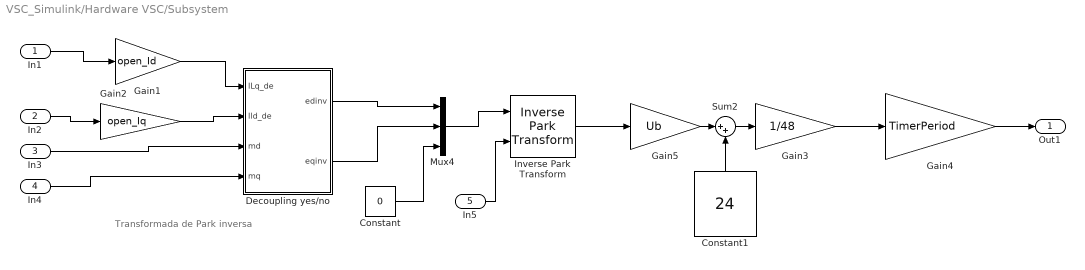
== system VSC_Simulink/Hardware VSC/Subsystem ==
  note: Transformada de Park inversa
  In1 : Inport
  In2 : Inport  Port=2
  In3 : Inport  Port=3
  In4 : Inport  Port=4
  In5 : Inport  Port=5
  Constant : Constant  Value=0  SampleTime=-1
  Constant1 : Constant  Value=24  SampleTime=-1
  Decoupling yes/no : Subsystem
  Gain1 : Gain  Gain=open_Id
  Gain2 : Gain  Gain=open_Iq
  Gain3 : Gain  Gain=1/48
  Gain4 : Gain  Gain=TimerPeriod
  Gain5 : Gain  Gain=Ub
  Inverse Park Transform : eeTransforms/Inverse Park Transform  AxisAlignment=Q-axis  PowerInvariant=on
      settings: SourceProductName=Simscape Electrical
  Mux4 : Mux  Inputs=3
  Sum2 : Sum  Inputs=|++
  Out1 : Outport  VectorParamsAs1DForOutWhenUnconnected=off
  wires:
  In5/1 -> Inverse Park Transform/2
  In3/1 -> Decoupling yes/no/3(md)
  In4/1 -> Decoupling yes/no/4(mq)
  In1/1 -> Gain1/1
  In2/1 -> Gain2/1
  Constant1/1 -> Sum2/2
  Sum2/1 -> Gain3/1
  Mux4/1 -> Inverse Park Transform/1
  Gain5/1 -> Sum2/1
  Inverse Park Transform/1 -> Gain5/1
  Decoupling yes/no/1(edinv) -> Mux4/1
  Decoupling yes/no/2(eqinv) -> Mux4/2
  Gain3/1 -> Gain4/1
  Gain4/1 -> Out1/1
  Constant/1 -> Mux4/3
  Gain1/1 -> Decoupling yes/no/1(ILq_de)
  Gain2/1 -> Decoupling yes/no/2(Ild_de)

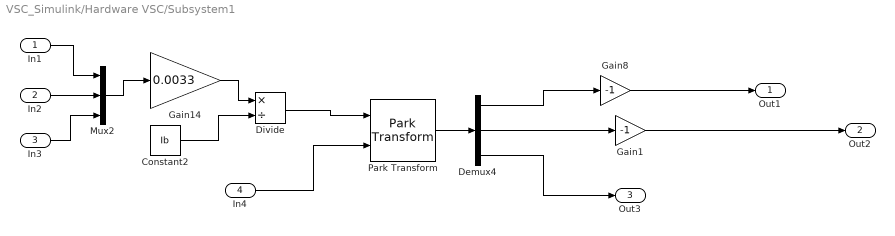
== system VSC_Simulink/Hardware VSC/Subsystem1 ==
  In1 : Inport
  In2 : Inport  Port=2
  In3 : Inport  Port=3
  In4 : Inport  Port=4
  Constant2 : Constant  Value=Ib  SampleTime=-1
  Demux4 : Demux  Outputs=3
  Divide : Product  Inputs=*/
  Gain1 : Gain  Gain=-1
  Gain14 : Gain  Gain=0.0033
  Gain8 : Gain  Gain=-1
  Mux2 : Mux  Inputs=3
  Park Transform : eeTransforms/Park Transform  AxisAlignment=Q-axis  PowerInvariant=on
      settings: SourceProductName=Simscape Electrical
  Out1 : Outport  VectorParamsAs1DForOutWhenUnconnected=off
  Out2 : Outport  Port=2  VectorParamsAs1DForOutWhenUnconnected=off
  Out3 : Outport  Port=3  VectorParamsAs1DForOutWhenUnconnected=off
  wires:
  Gain1/1 -> Out2/1
  Gain8/1 -> Out1/1
  Demux4/1 -> Gain8/1
  In2/1 -> Mux2/2
  Demux4/2 -> Gain1/1
  Demux4/3 -> Out3/1
  Gain14/1 -> Divide/1
  Mux2/1 -> Gain14/1
  In1/1 -> Mux2/1
  In4/1 -> Park Transform/2
  Constant2/1 -> Divide/2
  In3/1 -> Mux2/3
  Divide/1 -> Park Transform/1
  Park Transform/1 -> Demux4/1

== system VSC_Simulink/Hardware VSC/Subsystem2 ==
  In1 : Inport
  In2 : Inport  Port=2
  In3 : Inport  Port=3
  In4 : Inport  Port=4
  Sum : Sum  Inputs=|+-
  Sum1 : Sum  Inputs=|+-
  Out1 : Outport  VectorParamsAs1DForOutWhenUnconnected=off
  Out2 : Outport  Port=2  VectorParamsAs1DForOutWhenUnconnected=off
  wires:
  Sum/1 -> Out1/1
  In1/1 -> Sum/1
  In4/1 -> Sum1/2
  In3/1 -> Sum1/1
  Sum1/1 -> Out2/1
  In2/1 -> Sum/2

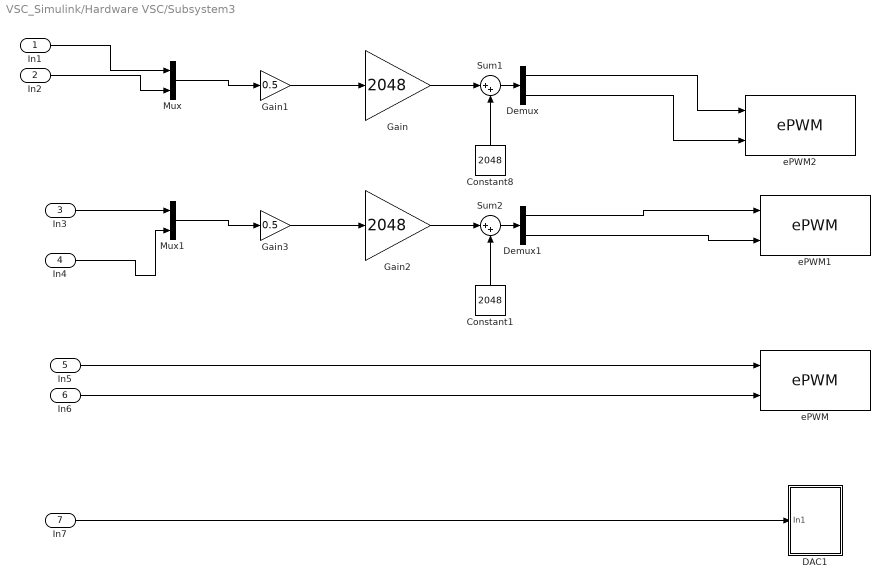
== system VSC_Simulink/Hardware VSC/Subsystem3 ==
  In1 : Inport
  In2 : Inport  Port=2
  In3 : Inport  Port=3
  In4 : Inport  Port=4
  In5 : Inport  Port=5
  In6 : Inport  Port=6
  In7 : Inport  Port=7
  Constant1 : Constant  Value=2048  SampleTime=-1
  Constant8 : Constant  Value=2048  SampleTime=-1
  DAC1 : Subsystem
  Demux : Demux  Outputs=2
  Demux1 : Demux  Outputs=2
  Gain : Gain  Gain=2048
  Gain1 : Gain  Gain=0.5
  Gain2 : Gain  Gain=2048
  Gain3 : Gain  Gain=0.5
  Mux : Mux  Inputs=2
  Mux1 : Mux  Inputs=2
  Sum1 : Sum  Inputs=|++
  Sum2 : Sum  Inputs=|++
  ePWM : c2802xlib/ePWM  useModule=ePWM3  ePWMxLINKTBPRD=Not Linked  periodUnits=Clock cycles  timerSource=Specify via dialog  timerPeriod_clk=TimerPeriod  timerPeriod_sec=0.0001  tbshadow=Counter equals to zero  countingMode=Up-Down  phaseActiveEnable=Disable  phaseDirection=Count down after sync  phaseActive=0  synchronizationEnable=off  dcaevt1Sync=off  dcbevt1Sync=off  synchronizationOption=Disable  clockPrescale=1  HSclockPrescale=1  enswap=off  ePWMxAStatus=on  ePWMxAactionLogic1=Set  ePWMxAactionLogic2=Clear  ePWMxAactionLogic3=Clear  ePWMxAactionLogic4=Set  ePWMxAactionLogic5=Do nothing  ePWMxAactionLogic6=Do nothing  ePWMxALoadMode=Load on counter equals to zero (CTR=Zero)  ePWMxACSFenable=off  ePWMxACSFvalue=Forcing disable  ePWMxASFreload=Zero  ePWMxBStatus=on  ePWMxBactionLogic1=Set  ePWMxBactionLogic2=Clear  ePWMxBactionLogic3=Do nothing  ePWMxBactionLogic4=Do nothing  ePWMxBactionLogic5=Clear  ePWMxBactionLogic6=Set  ePWMxBLoadMode=Load on counter equals to zero (CTR=Zero)  ePWMxBCSFenable=off  ePWMxBCSFvalue=Forcing disable  ePWMxBSFreload=Zero  ePWNxBOutWay=off  ePWMxLINKCMPA=Not Linked  CMPAUnits=Clock cycles  CMPASource=Input port  CMPAValue_per=50  CMPAValue_clk=0  enCMPAshadow=Counter equals to zero  ePWMxLINKCMPB=Not Linked  CMPBUnits=Clock cycles  CMPBSource=Input port  CMPBValue_per=50  CMPBValue_clk=0  enCMPBshadow=Counter equals to zero  ePWMxLINKCMPC=Not Linked  CMPCUnits=Clock cycles  CMPCSource=Specify via dialog  CMPCValue_per=50  CMPCValue_clk=0  enCMPCshadow=Counter equals to zero  ePWMxLINKCMPD=Not Linked  CMPDUnits=Clock cycles  CMPDSource=Specify via dialog  CMPDValue_per=50  CMPDValue_clk=0  enCMPDshadow=Counter equals to zero  enableDBePWMxA=off  enableDBePWMxB=off  enhalfcycle=off  DBpolarity=Active high (AH)  DBedgeDelay=Positive  DBSource_ePWMxA=ePWMxA  DBSource_ePWMxB=ePWMxA  DBperiodSource=Specify via dialog  REDperiod=0  FEDperiod=0  adcstartModuleA=off  adcrequestEventA=Third event  adcstartEventA=Digital Compare Module A Event 1 start of conversion (DCAEVT1.soc)  adcstartEventA_type2=Counter equals to period (CTR=PRD)  adcstartModuleB=off  adcrequestEventB=Third event  adcstartEventB=Counter equals to zero (CTR=Zero)  adcstartEventB_type2=Counter equals to period (CTR=PRD)  intEn=off  intPrd=First event  intSel=Counter equals to zero (CTR=Zero)  intSel_type2=Counter equals to zero (CTR=Zero)  hrpe=off  enHRPWM=off  HRPWM_LoadMode=Counter equals to period (CTR=PRD)  HRPWM_CTLMode=Duty or Period control mode  HRPWM_EDGMode=Both edge  hrpeb=off  enHRPWMB=off  HRPWM_LoadModeB=Counter equals to zero (CTR=ZERO)  HRPWM_CTLModeB=Duty or Period control mode  HRPWM_EDGModeB=Both edge  enSFO=on  enautoconv=on  chopperEnable=off  chopperFrequency=1  chopperFirstwidth=1  chopperDuty=12.5%  tripZonesource=Specify via dialog  tzselOSHT1=off  tzselOSHT2=off  tzselOSHT3=off  tzselOSHDCAEV1=off  tzselOSHDCBEV1=off  tzselCBC1=off  tzselCBC2=off  tzselCBC3=off  tzselCBCDCAEV2=off  tzselCBCDCBEV2=off  tzselOSHT4=off  tzselOSHT5=off  tzselOSHT6=off  tzselCBC4=off  tzselCBC5=off  tzselCBC6=off  enTzOstIntr=off  enTzCbcIntr=off  enTzDCAEVT1Intr=off  enTzDCAEVT2Intr=off  enTzDCBEVT1Intr=off  enTzDCBEVT2Intr=off  ePWMxAforced=No action  ePWMxBforced=No action  DCAEVT1forced=No action  DCBEVT1forced=No action  DCAEVT2forced=No action  DCBEVT2forced=No action  dcah=Trip Zone 1 input (TZ1)  dcal=Trip Zone 2 input (TZ2)  dcbh=Trip Zone 1 input (TZ1)  dcbl=Trip Zone 2 input (TZ2)  dcah_type2=GPTRIP1SEL/(TZ1)  dcal_type2=GPTRIP2SEL/(TZ2)  dcbh_type2=GPTRIP1SEL/(TZ1)  dcbl_type2=GPTRIP2SEL/(TZ2)  gendcaevt1=Event disabled  gendcaevt2=Event disabled  gendcbevt1=Event disabled  gendcbevt2=Event disabled  dcaevt1src=DCAEVT1 with sync  dcaevt2src=DCAEVT2 with sync  dcbevt1src=DCBEVT1 with sync  dcbevt2src=DCBEVT2 with sync  pulsesel=Counter equals to zero (CTR=Zero)  blankinv=off  blankoffset=0  blankwidth=0  evsrcsel=Filtered version of DCAEVT1 (DCAEVT1FILT)  encape=off  PwmType=C2000_Type4
      settings: SourceProductName=Embedded Coder Support Package for Texas Instruments C2000 Processors
  ePWM1 : c2802xlib/ePWM  useModule=ePWM2  ePWMxLINKTBPRD=Not Linked  periodUnits=Clock cycles  timerSource=Specify via dialog  timerPeriod_clk=TimerPeriod  timerPeriod_sec=0.0001  tbshadow=Counter equals to zero  countingMode=Up-Down  phaseActiveEnable=Disable  phaseDirection=Count down after sync  phaseActive=0  synchronizationEnable=off  dcaevt1Sync=off  dcbevt1Sync=off  synchronizationOption=Disable  clockPrescale=1  HSclockPrescale=1  enswap=off  ePWMxAStatus=on  ePWMxAactionLogic1=Set  ePWMxAactionLogic2=Clear  ePWMxAactionLogic3=Clear  ePWMxAactionLogic4=Set  ePWMxAactionLogic5=Do nothing  ePWMxAactionLogic6=Do nothing  ePWMxALoadMode=Load on counter equals to zero (CTR=Zero)  ePWMxACSFenable=off  ePWMxACSFvalue=Forcing disable  ePWMxASFreload=Zero  ePWMxBStatus=on  ePWMxBactionLogic1=Set  ePWMxBactionLogic2=Clear  ePWMxBactionLogic3=Do nothing  ePWMxBactionLogic4=Do nothing  ePWMxBactionLogic5=Clear  ePWMxBactionLogic6=Set  ePWMxBLoadMode=Load on counter equals to zero (CTR=Zero)  ePWMxBCSFenable=off  ePWMxBCSFvalue=Forcing disable  ePWMxBSFreload=Zero  ePWNxBOutWay=off  ePWMxLINKCMPA=Not Linked  CMPAUnits=Clock cycles  CMPASource=Input port  CMPAValue_per=50  CMPAValue_clk=0  enCMPAshadow=Counter equals to zero  ePWMxLINKCMPB=Not Linked  CMPBUnits=Clock cycles  CMPBSource=Input port  CMPBValue_per=50  CMPBValue_clk=0  enCMPBshadow=Counter equals to zero  ePWMxLINKCMPC=Not Linked  CMPCUnits=Clock cycles  CMPCSource=Specify via dialog  CMPCValue_per=50  CMPCValue_clk=0  enCMPCshadow=Counter equals to zero  ePWMxLINKCMPD=Not Linked  CMPDUnits=Clock cycles  CMPDSource=Specify via dialog  CMPDValue_per=50  CMPDValue_clk=0  enCMPDshadow=Counter equals to zero  enableDBePWMxA=off  enableDBePWMxB=off  enhalfcycle=off  DBpolarity=Active high (AH)  DBedgeDelay=Positive  DBSource_ePWMxA=ePWMxA  DBSource_ePWMxB=ePWMxA  DBperiodSource=Specify via dialog  REDperiod=0  FEDperiod=0  adcstartModuleA=off  adcrequestEventA=First event  adcstartEventA=Digital Compare Module A Event 1 start of conversion (DCAEVT1.soc)  adcstartEventA_type2=Digital Compare Module A Event 1 start of conversion (DCAEVT1.soc)  adcstartModuleB=off  adcrequestEventB=First event  adcstartEventB=Counter equals to zero (CTR=Zero)  adcstartEventB_type2=Counter equals to zero (CTR=Zero)  intEn=off  intPrd=First event  intSel=Counter equals to zero (CTR=Zero)  intSel_type2=Counter equals to zero (CTR=Zero)  hrpe=off  enHRPWM=off  HRPWM_LoadMode=Counter equals to period (CTR=PRD)  HRPWM_CTLMode=Duty or Period control mode  HRPWM_EDGMode=Both edge  hrpeb=off  enHRPWMB=off  HRPWM_LoadModeB=Counter equals to zero (CTR=ZERO)  HRPWM_CTLModeB=Duty or Period control mode  HRPWM_EDGModeB=Both edge  enSFO=on  enautoconv=on  chopperEnable=off  chopperFrequency=1  chopperFirstwidth=1  chopperDuty=12.5%  tripZonesource=Specify via dialog  tzselOSHT1=off  tzselOSHT2=off  tzselOSHT3=off  tzselOSHDCAEV1=off  tzselOSHDCBEV1=off  tzselCBC1=off  tzselCBC2=off  tzselCBC3=off  tzselCBCDCAEV2=off  tzselCBCDCBEV2=off  tzselOSHT4=off  tzselOSHT5=off  tzselOSHT6=off  tzselCBC4=off  tzselCBC5=off  tzselCBC6=off  enTzOstIntr=off  enTzCbcIntr=off  enTzDCAEVT1Intr=off  enTzDCAEVT2Intr=off  enTzDCBEVT1Intr=off  enTzDCBEVT2Intr=off  ePWMxAforced=No action  ePWMxBforced=No action  DCAEVT1forced=No action  DCBEVT1forced=No action  DCAEVT2forced=No action  DCBEVT2forced=No action  dcah=Trip Zone 1 input (TZ1)  dcal=Trip Zone 2 input (TZ2)  dcbh=Trip Zone 1 input (TZ1)  dcbl=Trip Zone 2 input (TZ2)  dcah_type2=GPTRIP1SEL/(TZ1)  dcal_type2=GPTRIP2SEL/(TZ2)  dcbh_type2=GPTRIP1SEL/(TZ1)  dcbl_type2=GPTRIP2SEL/(TZ2)  gendcaevt1=Event disabled  gendcaevt2=Event disabled  gendcbevt1=Event disabled  gendcbevt2=Event disabled  dcaevt1src=DCAEVT1 with sync  dcaevt2src=DCAEVT2 with sync  dcbevt1src=DCBEVT1 with sync  dcbevt2src=DCBEVT2 with sync  pulsesel=Counter equals to zero (CTR=Zero)  blankinv=off  blankoffset=0  blankwidth=0  evsrcsel=Filtered version of DCAEVT1 (DCAEVT1FILT)  encape=off  PwmType=C2000_Type4
      settings: SourceProductName=Embedded Coder Support Package for Texas Instruments C2000 Processors
  ePWM2 : c2802xlib/ePWM  useModule=ePWM1  ePWMxLINKTBPRD=Not Linked  periodUnits=Clock cycles  timerSource=Specify via dialog  timerPeriod_clk=TimerPeriod  timerPeriod_sec=0.0001  tbshadow=Counter equals to zero  countingMode=Up-Down  phaseActiveEnable=Disable  phaseDirection=Count down after sync  phaseActive=0  synchronizationEnable=off  dcaevt1Sync=off  dcbevt1Sync=off  synchronizationOption=Disable  clockPrescale=1  HSclockPrescale=1  enswap=off  ePWMxAStatus=on  ePWMxAactionLogic1=Set  ePWMxAactionLogic2=Clear  ePWMxAactionLogic3=Clear  ePWMxAactionLogic4=Set  ePWMxAactionLogic5=Do nothing  ePWMxAactionLogic6=Do nothing  ePWMxALoadMode=Load on counter equals to zero (CTR=Zero)  ePWMxACSFenable=off  ePWMxACSFvalue=Forcing disable  ePWMxASFreload=Zero  ePWMxBStatus=on  ePWMxBactionLogic1=Set  ePWMxBactionLogic2=Clear  ePWMxBactionLogic3=Do nothing  ePWMxBactionLogic4=Do nothing  ePWMxBactionLogic5=Clear  ePWMxBactionLogic6=Set  ePWMxBLoadMode=Load on counter equals to zero (CTR=Zero)  ePWMxBCSFenable=off  ePWMxBCSFvalue=Forcing disable  ePWMxBSFreload=Zero  ePWNxBOutWay=off  ePWMxLINKCMPA=Not Linked  CMPAUnits=Clock cycles  CMPASource=Input port  CMPAValue_per=50  CMPAValue_clk=0  enCMPAshadow=Counter equals to zero  ePWMxLINKCMPB=Not Linked  CMPBUnits=Clock cycles  CMPBSource=Input port  CMPBValue_per=50  CMPBValue_clk=0  enCMPBshadow=Counter equals to zero  ePWMxLINKCMPC=Not Linked  CMPCUnits=Clock cycles  CMPCSource=Specify via dialog  CMPCValue_per=50  CMPCValue_clk=0  enCMPCshadow=Counter equals to zero  ePWMxLINKCMPD=Not Linked  CMPDUnits=Clock cycles  CMPDSource=Specify via dialog  CMPDValue_per=50  CMPDValue_clk=0  enCMPDshadow=Counter equals to zero  enableDBePWMxA=off  enableDBePWMxB=off  enhalfcycle=off  DBpolarity=Active high (AH)  DBedgeDelay=Positive  DBSource_ePWMxA=ePWMxA  DBSource_ePWMxB=ePWMxA  DBperiodSource=Specify via dialog  REDperiod=0  FEDperiod=0  adcstartModuleA=off  adcrequestEventA=First event  adcstartEventA=Digital Compare Module A Event 1 start of conversion (DCAEVT1.soc)  adcstartEventA_type2=Digital Compare Module A Event 1 start of conversion (DCAEVT1.soc)  adcstartModuleB=off  adcrequestEventB=First event  adcstartEventB=Counter equals to zero (CTR=Zero)  adcstartEventB_type2=Counter equals to zero (CTR=Zero)  intEn=off  intPrd=First event  intSel=Counter equals to zero (CTR=Zero)  intSel_type2=Counter equals to zero (CTR=Zero)  hrpe=off  enHRPWM=off  HRPWM_LoadMode=Counter equals to period (CTR=PRD)  HRPWM_CTLMode=Duty or Period control mode  HRPWM_EDGMode=Both edge  hrpeb=off  enHRPWMB=off  HRPWM_LoadModeB=Counter equals to zero (CTR=ZERO)  HRPWM_CTLModeB=Duty or Period control mode  HRPWM_EDGModeB=Both edge  enSFO=on  enautoconv=on  chopperEnable=off  chopperFrequency=1  chopperFirstwidth=1  chopperDuty=12.5%  tripZonesource=Specify via dialog  tzselOSHT1=off  tzselOSHT2=off  tzselOSHT3=off  tzselOSHDCAEV1=off  tzselOSHDCBEV1=off  tzselCBC1=off  tzselCBC2=off  tzselCBC3=off  tzselCBCDCAEV2=off  tzselCBCDCBEV2=off  tzselOSHT4=off  tzselOSHT5=off  tzselOSHT6=off  tzselCBC4=off  tzselCBC5=off  tzselCBC6=off  enTzOstIntr=off  enTzCbcIntr=off  enTzDCAEVT1Intr=off  enTzDCAEVT2Intr=off  enTzDCBEVT1Intr=off  enTzDCBEVT2Intr=off  ePWMxAforced=No action  ePWMxBforced=No action  DCAEVT1forced=No action  DCBEVT1forced=No action  DCAEVT2forced=No action  DCBEVT2forced=No action  dcah=Trip Zone 1 input (TZ1)  dcal=Trip Zone 2 input (TZ2)  dcbh=Trip Zone 1 input (TZ1)  dcbl=Trip Zone 2 input (TZ2)  dcah_type2=GPTRIP1SEL/(TZ1)  dcal_type2=GPTRIP2SEL/(TZ2)  dcbh_type2=GPTRIP1SEL/(TZ1)  dcbl_type2=GPTRIP2SEL/(TZ2)  gendcaevt1=Event disabled  gendcaevt2=Event disabled  gendcbevt1=Event disabled  gendcbevt2=Event disabled  dcaevt1src=DCAEVT1 with sync  dcaevt2src=DCAEVT2 with sync  dcbevt1src=DCBEVT1 with sync  dcbevt2src=DCBEVT2 with sync  pulsesel=Counter equals to zero (CTR=Zero)  blankinv=off  blankoffset=0  blankwidth=0  evsrcsel=Filtered version of DCAEVT1 (DCAEVT1FILT)  encape=off  PwmType=C2000_Type4
      settings: SourceProductName=Embedded Coder Support Package for Texas Instruments C2000 Processors
  wires:
  In7/1 -> DAC1/1(In1)
  In6/1 -> ePWM/2
  Mux1/1 -> Gain3/1
  Constant1/1 -> Sum2/2
  Gain2/1 -> Sum2/1
  Gain3/1 -> Gain2/1
  Sum2/1 -> Demux1/1
  In2/1 -> Mux/2
  Sum1/1 -> Demux/1
  Gain1/1 -> Gain/1
  Gain/1 -> Sum1/1
  Constant8/1 -> Sum1/2
  Mux/1 -> Gain1/1
  In4/1 -> Mux1/2
  In3/1 -> Mux1/1
  In5/1 -> ePWM/1
  Demux1/2 -> ePWM1/2
  Demux1/1 -> ePWM1/1
  Demux/1 -> ePWM2/1
  Demux/2 -> ePWM2/2
  In1/1 -> Mux/1
